simulink model "process_ss"  (R2018b)
settings: Solver=VariableStepAuto  StartTime=0.0  StopTime=500  RelTol=1e-3
settings Model: Creator=jh2044  LastModifiedBy=gv281
settings DataIOCC: SaveFinalState=on

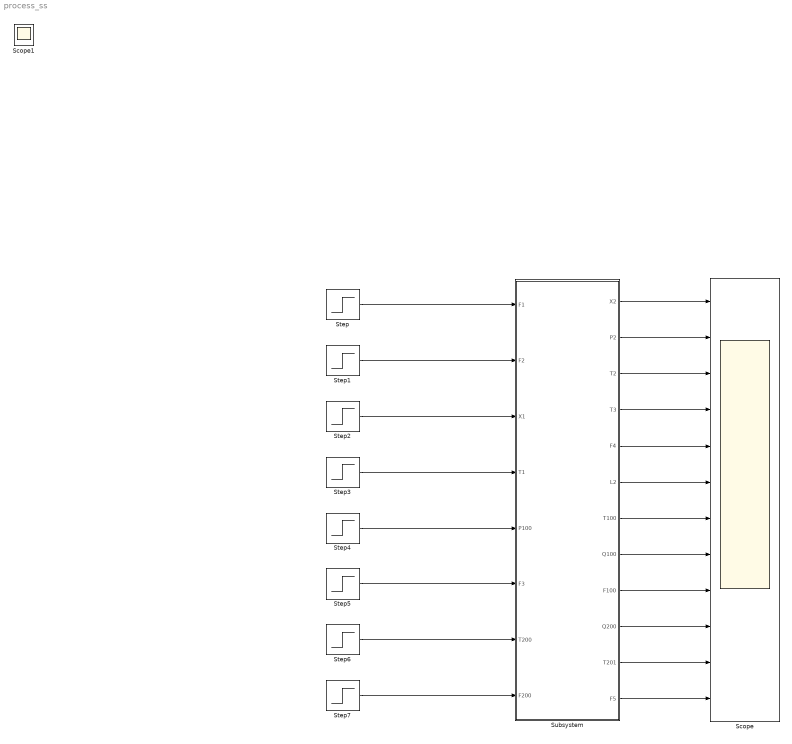
== system process_ss ==
  Scope : Scope  NumInputPorts=12
  Step : Step  After=10  SampleTime=0
  Step1 : Step  After=2  SampleTime=0
  Step2 : Step  After=5  SampleTime=0
  Step3 : Step  After=40  SampleTime=0
  Step4 : Step  After=194.7  SampleTime=0
  Step5 : Step  After=50  SampleTime=0
  Step6 : Step  After=25  SampleTime=0
  Step7 : Step  Before=1  After=208  SampleTime=0
  Subsystem : Subsystem
  Scope1 : Scope
  wires:
  Step/1 -> Subsystem/1(F1)
  Step1/1 -> Subsystem/2(F2)
  Step2/1 -> Subsystem/3(X1)
  Step3/1 -> Subsystem/4(T1)
  Step4/1 -> Subsystem/5(P100)
  Step5/1 -> Subsystem/6(F3)
  Step6/1 -> Subsystem/7(T200)
  Step7/1 -> Subsystem/8(F200)
  Subsystem/1(X2) -> Scope/1
  Subsystem/2(P2) -> Scope/2
  Subsystem/3(T2) -> Scope/3
  Subsystem/4(T3) -> Scope/4
  Subsystem/5(F4) -> Scope/5
  Subsystem/6(L2) -> Scope/6
  Subsystem/7(T100) -> Scope/7
  Subsystem/8(Q100) -> Scope/8
  Subsystem/9(F100) -> Scope/9
  Subsystem/10(Q200) -> Scope/10
  Subsystem/11(T201) -> Scope/11
  Subsystem/12(F5) -> Scope/12

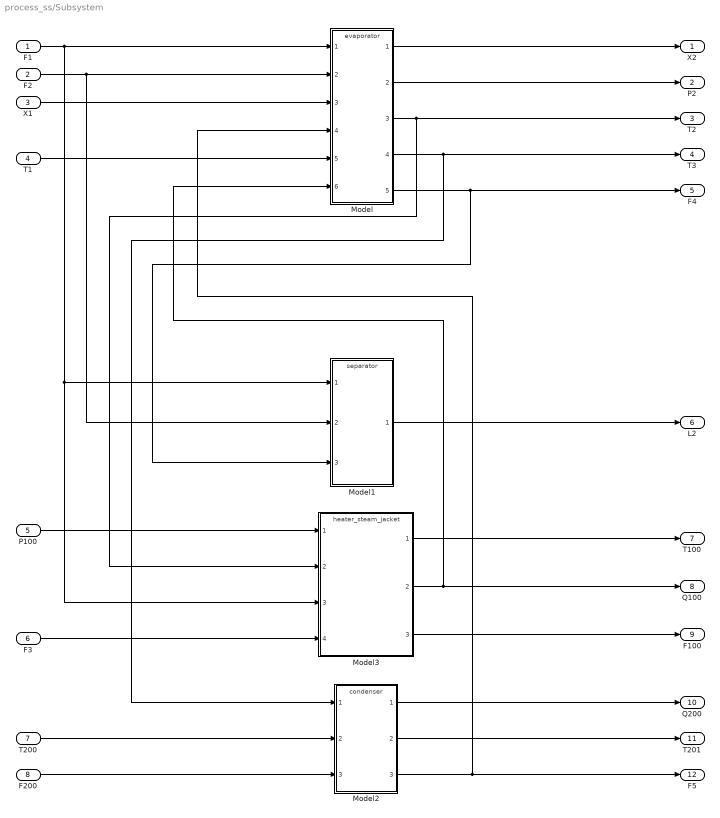
== system process_ss/Subsystem ==
  F1 : Inport
  F2 : Inport  Port=2
  X1 : Inport  Port=3
  T1 : Inport  Port=4
  P100 : Inport  Port=5
  F3 : Inport  Port=6
  T200 : Inport  Port=7
  F200 : Inport  Port=8
  Model : ModelReference  ModelNameDialog=evaporator  SimulationMode=Normal  ModelReferenceVersion=1.9
  Model1 : ModelReference  ModelNameDialog=separator  SimulationMode=Normal  ModelReferenceVersion=1.3
  Model2 : ModelReference  ModelNameDialog=condenser  SimulationMode=Normal  ModelReferenceVersion=1.15
  Model3 : ModelReference  ModelNameDialog=heater_steam_jacket.slx  SimulationMode=Normal  ModelReferenceVersion=1.5
  X2 : Outport
  P2 : Outport  Port=2
  T2 : Outport  Port=3
  T3 : Outport  Port=4
  F4 : Outport  Port=5
  L2 : Outport  Port=6
  T100 : Outport  Port=7
  Q100 : Outport  Port=8
  F100 : Outport  Port=9
  Q200 : Outport  Port=10
  T201 : Outport  Port=11
  F5 : Outport  Port=12
  wires:
  F3/1 -> Model3/4
  Model1/1 -> L2/1
  Model3/1 -> T100/1
  Model2/1 -> Q200/1
  X1/1 -> Model/3
  T1/1 -> Model/5
  Model3/2 -> Q100/1, Model/6
  Model2/2 -> T201/1
  Model/1 -> X2/1
  T200/1 -> Model2/2
  Model/5 -> F4/1, Model1/3
  Model/2 -> P2/1
  P100/1 -> Model3/1
  Model2/3 -> F5/1, Model/4
  Model/4 -> T3/1, Model2/1
  F200/1 -> Model2/3
  Model3/3 -> F100/1
  F2/1 -> Model1/2, Model/2
  Model/3 -> T2/1, Model3/2
  F1/1 -> Model3/3, Model1/1, Model/1
